simulink model "testSignalGenerator"  (R2018b)
settings: Solver=VariableStepAuto  StartTime=0.0  StopTime=40  RelTol=1e-3
values from neighbouring files (symbols this model uses):
  Ts = 0.05    [dataToCSV.m]
settings Model: Creator=Marko  LastModifiedBy=mandicluka

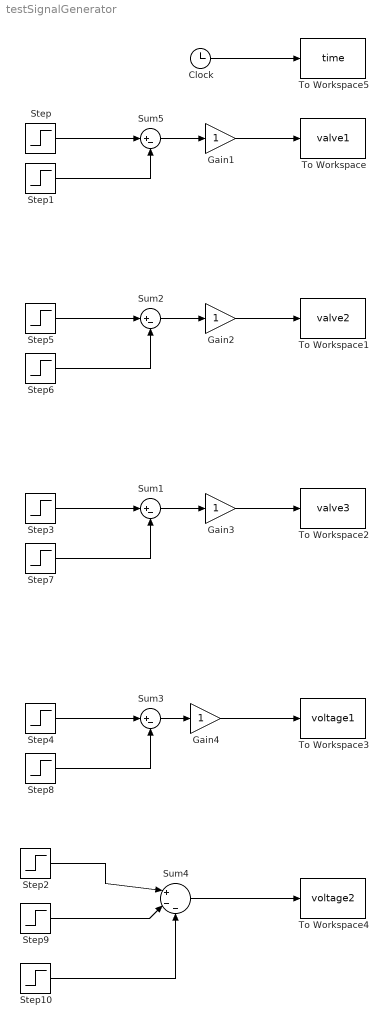
== system testSignalGenerator ==
  Clock : Clock
  Gain{1..4} (4 alike) : Gain
  Step : Step  Time=21  After=0.005  SampleTime=0
  Step1 : Step  Time=25  After=0.005  SampleTime=0
  Step10 : Step  Time=55  After=120  SampleTime=0
  Step2 : Step  Time=0  After=180  SampleTime=0
  Step3 : Step  Time=11  After=0.005  SampleTime=0
  Step4 : Step  Time=31  After=250  SampleTime=0
  Step5 : Step  Time=0  After=0.005  SampleTime=0
  Step6 : Step  Time=10  After=0.005  SampleTime=0
  Step7 : Step  Time=20  After=0.005  SampleTime=0
  Step8 : Step  Time=50  After=250  SampleTime=0
  Step9 : Step  Time=7  After=180  SampleTime=0
  Sum{1..3,5} (4 alike) : Sum  Inputs=|+-
  Sum4 : Sum  Inputs=|+--
  To Workspace : ToWorkspace  VariableName=valve1  SampleTime=Ts
      settings: Save2DSignal=2-D array (concatenate along first dimension)
  To Workspace1 : ToWorkspace  VariableName=valve2  SampleTime=Ts
      settings: Save2DSignal=2-D array (concatenate along first dimension)
  To Workspace2 : ToWorkspace  VariableName=valve3  SampleTime=Ts
      settings: Save2DSignal=2-D array (concatenate along first dimension)
  To Workspace3 : ToWorkspace  VariableName=voltage1  SampleTime=Ts
      settings: Save2DSignal=2-D array (concatenate along first dimension)
  To Workspace4 : ToWorkspace  VariableName=voltage2  SampleTime=Ts
      settings: Save2DSignal=2-D array (concatenate along first dimension)
  To Workspace5 : ToWorkspace  VariableName=time  SampleTime=Ts
      settings: Save2DSignal=2-D array (concatenate along first dimension)
  wires:
  Step9/1 -> Sum4/2
  Sum3/1 -> Gain4/1
  Step3/1 -> Sum1/1
  Step6/1 -> Sum2/2
  Step7/1 -> Sum1/2
  Step8/1 -> Sum3/2
  Sum2/1 -> Gain2/1
  Step/1 -> Sum5/1
  Step10/1 -> Sum4/3
  Step5/1 -> Sum2/1
  Step2/1 -> Sum4/1
  Step4/1 -> Sum3/1
  Sum5/1 -> Gain1/1
  Sum1/1 -> Gain3/1
  Step1/1 -> Sum5/2
  Gain1/1 -> To Workspace/1
  Gain2/1 -> To Workspace1/1
  Gain3/1 -> To Workspace2/1
  Gain4/1 -> To Workspace3/1
  Sum4/1 -> To Workspace4/1
  Clock/1 -> To Workspace5/1
